simulink model "TEST_TCP"  (R2022b)
settings: Solver=FixedStepAuto  StartTime=0.0  StopTime=inf  FixedStep=1e-3  RelTol=1e-3  EnableMultiTasking=on
undefined symbols (not defined in the file or in its folder): angular, CIRCUIT, CLTF_DAMP, CLTF_FREQ, CLTF_GAIN, CONTROL, CONTROL_INI, DiscIntNeverNeededParam, INPUT, linear, MCP3201, MD25, MODEL, MODEL_INI, mpcstate, MPU60X0, MPU9250, MSG, NAV_MPC_CONTROL, OUTPUT, RCRX, SAMPLING_TIME, SYSID_INPUT, VL6180X
libraries: raspberrypiCommlib x156, simulink x86, dspsigattribs x14, raspberrypiNetworklib x13, embedlinuxBasiclib x9, ctrlSharedLib x2, ros2lib x2, mpclib x1, vrlib x1, sldrtlib x1
(part 5 of 17)

== system TEST_TCP/HARDWARE/SENSORS/IMU MPU60X0_SPI/READ FIFO ==
  Enable : EnablePort
  Constant2 : Constant  Commented=on  Value=bin2dec('01000100');  OutDataTypeStr=uint8  SampleTime=SAMPLING_TIME
  Constant3 : Constant  Value=MPU60X0.ACCEL_SSF  SampleTime=SAMPLING_TIME
  Constant4 : Constant  Value=MPU60X0.GYRO_SSF  SampleTime=SAMPLING_TIME
  Constant7 : Constant  Value=MPU60X0.FIFO_LENGTH  OutDataTypeStr=uint8  SampleTime=SAMPLING_TIME
  Data Store Read : DataStoreRead  DataStoreName=CONTROL  DataStoreElements=CONTROL_BUS.INPUT.IMU.ACCEL_MEAN(:,:)#CONTROL_BUS.INPUT.IMU.GYRO_MEAN(:,:)  IndexOptions=Index vector (dialog)  Indices=1  OutputSizes=1
  Data Store Read2 : DataStoreRead  DataStoreName=CONTROL  SampleTime=SAMPLING_TIME  IndexOptions=Index vector (dialog)  Indices=1  OutputSizes=1
  Data Store Write : DataStoreWrite  DataStoreName=CONTROL  IndexOptions=Index vector (dialog)  Indices=1  OutputSizes=1
  Data Store Write1 : DataStoreWrite  DataStoreName=MPU60X0_RAW_GYRO_MEAN  IndexOptions=Index vector (dialog)  Indices=1  OutputSizes=1
  Data Store Write2 : DataStoreWrite  DataStoreName=MPU60X0_RAW_ACCEL_MEAN  IndexOptions=Index vector (dialog)  Indices=1  OutputSizes=1
  Data Type Conversion : DataTypeConversion  OutDataTypeStr=double  SaturateOnIntegerOverflow=off  RndMeth=Floor
  Data Type Conversion4 : DataTypeConversion  OutDataTypeStr=int16  SaturateOnIntegerOverflow=off  RndMeth=Floor
  EVEN POSITIONS : Selector  InputPortWidth=uint8(12*MPU9250.FIFO_LENGTH)  IndexOptions=Index vector (dialog)  Indices=2:2:uint8(12*MPU9250.FIFO_LENGTH)  OutputSizes=1
  FIFO READ : Subsystem  mask{Register=MPU60X0.FIFO_R_W, n=12*MPU60X0.FIFO_LENGTH}
      mask prompts: Register "MPU9250 Register"; n "Data size (bytes)"
      mask DialogControl Control2 Prompt: (Add text here)
  FIFO RESET : raspberrypiCommlib/SPI Register Write  Priority=20  Commented=on  BoardProperty=Pi 3 Model B+  SSPin=SPI0_CE1  SPIModule=uint32(0)  Mode=Master  BusSpeed=1000000  Pin=SPI0_CE0  FirstBitToTransfer=Most significant bit (MSB)  ClockMode=3  BlockFunction=Write  RegisterAddress=MPU60X0.USER_CTRL  OutputDataType=int8  OutputDataLength=1
  FIFO_PROCESSING : MATLAB Function  Priority=30  TreatAsAtomicUnit=on
  Gain61 : Gain  Gain=2^8
  Mux : Mux
  ODD POSITIONS : Selector  InputPortWidth=uint8(12*MPU9250.FIFO_LENGTH)  IndexOptions=Index vector (dialog)  Indices=1:2:uint8(12*MPU9250.FIFO_LENGTH)  OutputSizes=1
  Sum61 : Sum  Inputs=|++
  To File : ToFile  Filename=BLACK_BOX_FIFO.mat  MatrixName=FIFO_LOG
  wires:
  Data Store Read/2 -> Mux/4
  Data Store Read/1 -> Mux/3
  FIFO_PROCESSING/5(GYRO_FIFO) -> Mux/2
  FIFO_PROCESSING/4(ACCEL_FIFO) -> Mux/1
  Constant4/1 -> FIFO_PROCESSING/5(GYRO_SSF)
  Constant3/1 -> FIFO_PROCESSING/4(ACCEL_SSF)
  Mux/1 -> Data Type Conversion/1
  Data Type Conversion/1 -> To File/1
  Data Type Conversion4/1 -> FIFO_PROCESSING/2(FIFO_DATA)
  FIFO READ/1(Out1) -> ODD POSITIONS/1, EVEN POSITIONS/1
  FIFO_PROCESSING/3(RAW_ACCEL_MEAN_OUT) -> Data Store Write2/1
  FIFO_PROCESSING/2(RAW_GYRO_MEAN_OUT) -> Data Store Write1/1
  Constant2/1 -> FIFO RESET/1
  Data Store Read2/1 -> FIFO_PROCESSING/1(CONTROL_IN)
  Sum61/1 -> Data Type Conversion4/1
  FIFO_PROCESSING/1(CONTROL_OUT) -> Data Store Write/1
  Constant7/1 -> FIFO_PROCESSING/3(FIFO_LENGTH)
  EVEN POSITIONS/1 -> Sum61/2
  Gain61/1 -> Sum61/1
  ODD POSITIONS/1 -> Gain61/1

== system TEST_TCP/HARDWARE/SENSORS/IMU MPU60X0_SPI/READ IMU ==
  Enable : EnablePort
  " LPF 3" : Subsystem
  " LPF 4" : Subsystem
  ACCELEROMETER : Subsystem  mask{REGISTER_ADDRESS=MPU60X0.ACCEL_XOUT_H, READ_FLAG=MPU60X0.READ_FLAG, N=6, Ts=MPU60X0.SAMPLING_TIME}
      mask prompts: REGISTER_ADDRESS "REGISTER ADDRESS"; READ_FLAG "READ FLAG"; N "DATA SIZE (BYTES)"; Ts "SAMPLING TIME (s)"
  Constant2 : Constant  Value=MPU60X0.ACCEL_CALIB  SampleTime=MPU60X0.SAMPLING_TIME
  Constant3 : Constant  Value=CONTROL_INI.PARAM.GRAVITY  SampleTime=MPU60X0.SAMPLING_TIME
  Constant4 : Constant  Value=MPU60X0.ALFA_CALIB  SampleTime=MPU60X0.SAMPLING_TIME
  Data Store Memory1 : DataStoreMemory  Priority=10  DataStoreName=MPU60X0_PITCH_OFFS  ReadBeforeWriteMsg=warning  WriteAfterWriteMsg=warning  WriteAfterReadMsg=warning  ShowAdditionalParam=off  OutDataTypeStr=double
  Data Store Memory5 : DataStoreMemory  Priority=10  DataStoreName=MPU60X0_ACCEL_OFFS  ReadBeforeWriteMsg=warning  WriteAfterWriteMsg=warning  WriteAfterReadMsg=warning  InitialValue=zeros(3,1)  ShowAdditionalParam=off  OutDataTypeStr=double
  Data Store Memory6 : DataStoreMemory  Priority=10  DataStoreName=MPU60X0_GYRO_OFFS  ReadBeforeWriteMsg=warning  WriteAfterWriteMsg=warning  WriteAfterReadMsg=warning  InitialValue=zeros(3,1)  ShowAdditionalParam=off  OutDataTypeStr=double
  Data Store Read : DataStoreRead  DataStoreName=CONTROL  SampleTime=MPU60X0.SAMPLING_TIME  DataStoreElements=CONTROL.STATE.VEHICLE_MODE  IndexOptions=Index vector (dialog)  Indices=1  OutputSizes=1
  Data Store Read1 : DataStoreRead  DataStoreName=MPU60X0_PITCH_OFFS  SampleTime=MPU60X0.SAMPLING_TIME  IndexOptions=Index vector (dialog)  Indices=1  OutputSizes=1
  Data Store Read6 : DataStoreRead  DataStoreName=MPU60X0_ACCEL_OFFS  SampleTime=MPU60X0.SAMPLING_TIME  IndexOptions=Index vector (dialog)  Indices=1  OutputSizes=1
  Data Store Read8 : DataStoreRead  DataStoreName=MPU60X0_GYRO_OFFS  SampleTime=MPU60X0.SAMPLING_TIME  IndexOptions=Index vector (dialog)  Indices=1  OutputSizes=1
  Data Store Read9 : DataStoreRead  DataStoreName=CONTROL  SampleTime=MPU60X0.SAMPLING_TIME  IndexOptions=Index vector (dialog)  Indices=1  OutputSizes=1
  Data Store Write3 : DataStoreWrite  DataStoreName=MPU60X0_ACCEL_OFFS  IndexOptions=Index vector (dialog)  Indices=1  OutputSizes=1
  Data Store Write4 : DataStoreWrite  DataStoreName=MPU60X0_GYRO_OFFS  IndexOptions=Index vector (dialog)  Indices=1  OutputSizes=1
  Data Store Write5 : DataStoreWrite  DataStoreName=CONTROL  IndexOptions=Index vector (dialog)  Indices=1  OutputSizes=1
  Data Type Conversion1 : DataTypeConversion  OutDataTypeStr=int16  SaturateOnIntegerOverflow=off  RndMeth=Floor
  Data Type Conversion2 : DataTypeConversion  OutDataTypeStr=double  SaturateOnIntegerOverflow=off  RndMeth=Floor
  Data Type Conversion3 : DataTypeConversion  OutDataTypeStr=double  SaturateOnIntegerOverflow=off  RndMeth=Floor
  Data Type Conversion4 : DataTypeConversion  OutDataTypeStr=int16  SaturateOnIntegerOverflow=off  RndMeth=Floor
  EVEN POSITIONS : Selector  InputPortWidth=uint8(6)  IndexOptions=Index vector (dialog)  Indices=2:2:uint8(6)  OutputSizes=1
  "EVEN POSITIONS  " : Selector  InputPortWidth=uint8(6)  IndexOptions=Index vector (dialog)  Indices=2:2:uint8(6)  OutputSizes=1
  FILTER POLE : Subsystem
  GRAVITY ROTATION : MATLAB Function  TreatAsAtomicUnit=on
  GYROSCOPE : Subsystem  mask{REGISTER_ADDRESS=MPU60X0.GYRO_XOUT_H, READ_FLAG=MPU60X0.READ_FLAG, N=6, Ts=MPU60X0.SAMPLING_TIME}
      mask prompts: REGISTER_ADDRESS "REGISTER ADDRESS"; READ_FLAG "READ FLAG"; N "DATA SIZE (BYTES)"; Ts "SAMPLING TIME (s)"
  Gain : Gain  Gain=CONTROL_INI.PARAM.GRAVITY/MPU60X0.ACCEL_SSF
  Gain1 : Gain  Gain=pi/MPU60X0.GYRO_SSF/180
  Gain4 : Gain  Gain=2^8
  Gain61 : Gain  Gain=2^8
  IMU CALIBRATION : MATLAB Function  Priority=30  TreatAsAtomicUnit=on
  LPF 1 : Subsystem
  "LPF 2 " : Subsystem
  MEAN FILTER : DiscreteFilter  Numerator=1/floor(SAMPLING_TIME*1000)*ones(1,floor(SAMPLING_TIME*1000))  Denominator=[1 zeros(1,floor(SAMPLING_TIME*1000)-1)]
  "MEAN FILTER " : DiscreteFilter  Numerator=1/floor(SAMPLING_TIME*1000)*ones(1,floor(SAMPLING_TIME*1000))  Denominator=[1 zeros(1,floor(SAMPLING_TIME*1000)-1)]
  ODD POSITIONS : Selector  InputPortWidth=uint8(6)  IndexOptions=Index vector (dialog)  Indices=1:2:uint8(6)  OutputSizes=1
  "ODD POSITIONS  " : Selector  InputPortWidth=uint8(6)  IndexOptions=Index vector (dialog)  Indices=1:2:uint8(6)  OutputSizes=1
  Sum4 : Sum  Inputs=|++
  Sum61 : Sum  Inputs=|++
  wires:
  ODD POSITIONS/1 -> Gain61/1
  EVEN POSITIONS/1 -> Sum61/2
  ACCELEROMETER/1(DATA_OUT) -> EVEN POSITIONS/1, ODD POSITIONS/1
  Sum61/1 -> Data Type Conversion4/1
  Gain61/1 -> Sum61/1
  Sum4/1 -> Data Type Conversion1/1
  Gain4/1 -> Sum4/1
  GYROSCOPE/1(DATA_OUT) -> "EVEN POSITIONS  "/1, "ODD POSITIONS  "/1
  "EVEN POSITIONS  "/1 -> Sum4/2
  "ODD POSITIONS  "/1 -> Gain4/1
  Data Type Conversion4/1 -> Data Type Conversion2/1
  Data Type Conversion1/1 -> Data Type Conversion3/1
  Data Type Conversion2/1 -> Gain/1
  Data Type Conversion3/1 -> Gain1/1
  Constant4/1 -> IMU CALIBRATION/11(ALFA_CALIB)
  Constant2/1 -> IMU CALIBRATION/10(ACCEL_CALIB)
  FILTER POLE/1(ALFA) -> " LPF 4"/2(ALFA), " LPF 3"/2(ALFA), LPF 1/2(ALFA), "LPF 2 "/2(ALFA)
  Gain1/1 -> "MEAN FILTER "/1, IMU CALIBRATION/6(GYRO), " LPF 3"/1(IN)
  LPF 1/1(OUT) -> IMU CALIBRATION/3(ACCEL_FILT)
  " LPF 3"/1(OUT) -> IMU CALIBRATION/7(GYRO_FILT)
  " LPF 4"/1(OUT) -> IMU CALIBRATION/9(GYRO_MEAN_FILT)
  Data Store Read9/1 -> IMU CALIBRATION/1(CONTROL_IN)
  "LPF 2 "/1(OUT) -> IMU CALIBRATION/5(ACCEL_MEAN_FILT)
  IMU CALIBRATION/3(GYRO_OFFS_OUT) -> Data Store Write4/1
  Data Store Read6/1 -> IMU CALIBRATION/12(ACCEL_OFFS_IN)
  IMU CALIBRATION/1(CONTROL) -> Data Store Write5/1
  MEAN FILTER/1 -> "LPF 2 "/1(IN), IMU CALIBRATION/4(ACCEL_MEAN)
  Data Store Read8/1 -> IMU CALIBRATION/13(GYRO_OFFS_IN)
  IMU CALIBRATION/2(ACCEL_OFFS_OUT) -> Data Store Write3/1
  "MEAN FILTER "/1 -> IMU CALIBRATION/8(GYRO_MEAN), " LPF 4"/1(IN)
  Gain/1 -> MEAN FILTER/1, IMU CALIBRATION/2(ACCEL), LPF 1/1(IN)
  Constant3/1 -> GRAVITY ROTATION/2(GRAVITY)
  Data Store Read1/1 -> GRAVITY ROTATION/1(PITCH_OFFSET)
  GRAVITY ROTATION/1(GRAVITY_VECTOR) -> IMU CALIBRATION/14(GRAVITY_VECTOR)
  Data Store Read/1 -> GRAVITY ROTATION/3(VEHICLE_MODE)

== system TEST_TCP/HARDWARE/SENSORS/IMU MPU60X0_SPI/READ TEMP ==
  Enable : EnablePort
  Bus Assignment : BusAssignment  AssignedSignals=INPUT.IMU.TEMP
  Constant1 : Constant  Value=MPU60X0.TEMP_SSF  SampleTime=MPU60X0.SAMPLING_TIME
  Constant2 : Constant  Value=MPU60X0.TEMP_OFFS  SampleTime=MPU60X0.SAMPLING_TIME
  Data Store Read1 : DataStoreRead  DataStoreName=CONTROL  SampleTime=MPU60X0.SAMPLING_TIME  IndexOptions=Index vector (dialog)  Indices=1  OutputSizes=1
  Data Store Read2 : DataStoreRead  DataStoreName=CONTROL  SampleTime=MPU60X0.SAMPLING_TIME  IndexOptions=Index vector (dialog)  Indices=1  OutputSizes=1
  Data Store Write : DataStoreWrite  DataStoreName=CONTROL  IndexOptions=Index vector (dialog)  Indices=1  OutputSizes=1
  Data Store Write1 : DataStoreWrite  DataStoreName=CONTROL  IndexOptions=Index vector (dialog)  Indices=1  OutputSizes=1
  Data Type Conversion3 : DataTypeConversion  OutDataTypeStr=int16  SaturateOnIntegerOverflow=off  RndMeth=Floor
  Demux : Demux  Outputs=2
  Gain61 : Gain  Gain=2^8
  IMU SCALING : MATLAB Function  Priority=40  TreatAsAtomicUnit=on
  Sum61 : Sum  Inputs=|++
  TEMP_READ : Subsystem  mask{REGISTER_ADDRESS=MPU60X0.TEMP_OUT_H, READ_FLAG=MPU60X0.READ_FLAG, N=2, Ts=MPU60X0.SAMPLING_TIME}
      mask prompts: REGISTER_ADDRESS "REGISTER ADDRESS"; READ_FLAG "READ FLAG"; N "DATA SIZE (BYTES)"; Ts "SAMPLING TIME (s)"
  wires:
  IMU SCALING/1(CONTROL_OUT) -> Data Store Write/1
  Demux/2 -> Sum61/2
  Sum61/1 -> Data Type Conversion3/1
  Bus Assignment/1 -> Data Store Write1/1
  Data Store Read1/1 -> Bus Assignment/1
  Gain61/1 -> Sum61/1
  Demux/1 -> Gain61/1
  Constant2/1 -> IMU SCALING/3(TEMP_OFFS)
  Data Type Conversion3/1 -> Bus Assignment/2
  Data Store Read2/1 -> IMU SCALING/1(CONTROL_IN)
  Constant1/1 -> IMU SCALING/2(TEMP_SSF)
  TEMP_READ/1(DATA_OUT) -> Demux/1

== system TEST_TCP/HARDWARE/SENSORS/IMU MPU60X0_SPI/WHO_AM_I ==
  Enable : EnablePort
  Display : Display
  MPU60X0_WHO_AM_I : Subsystem  Priority=10  mask{REGISTER_ADDRESS=MPU60X0.WHO_AM_I, READ_FLAG=MPU60X0.READ_FLAG, N=1, Ts=MPU60X0.SAMPLING_TIME}
      mask prompts: REGISTER_ADDRESS "REGISTER ADDRESS"; READ_FLAG "READ FLAG"; N "DATA SIZE (BYTES)"; Ts "SAMPLING TIME (s)"
  wires:
  MPU60X0_WHO_AM_I/1(DATA_OUT) -> Display/1

== system TEST_TCP/HARDWARE/SENSORS/WALL RANGE SENSOR/ANGLE AND DISTANCE COMPUTATION ==
  Data Store Read : DataStoreRead  DataStoreName=FRONT_DISTANCE  SampleTime=SAMPLING_TIME  IndexOptions=Index vector (dialog)  Indices=1  OutputSizes=1
  Data Store Read1 : DataStoreRead  DataStoreName=REAR_DISTANCE  IndexOptions=Index vector (dialog)  Indices=1  OutputSizes=1
  Data Store Read2 : DataStoreRead  DataStoreName=CONTROL  SampleTime=SAMPLING_TIME  IndexOptions=Index vector (dialog)  Indices=1  OutputSizes=1
  Data Store Write1 : DataStoreWrite  DataStoreName=CONTROL  IndexOptions=Index vector (dialog)  Indices=1  OutputSizes=1
  YAW_ANGLE_DISTANCE_COMPUTATION : MATLAB Function  TreatAsAtomicUnit=on
  wires:
  Data Store Read/1 -> YAW_ANGLE_DISTANCE_COMPUTATION/1(FRONT_DISTANCE)
  Data Store Read1/1 -> YAW_ANGLE_DISTANCE_COMPUTATION/2(REAR_DISTANCE)
  Data Store Read2/1 -> YAW_ANGLE_DISTANCE_COMPUTATION/3(CONTROL_IN)
  YAW_ANGLE_DISTANCE_COMPUTATION/1(CONTROL) -> Data Store Write1/1

== system TEST_TCP/HARDWARE/SENSORS/WALL RANGE SENSOR/VL6180X_I2C_FRONT ==
  Constant2 : Constant  Value=hex2dec('02')  OutDataTypeStr=uint8  SampleTime=SAMPLING_TIME
  Data Store Memory1 : DataStoreMemory  Priority=10  DataStoreName=VL6180X_COUNTER  ReadBeforeWriteMsg=warning  WriteAfterWriteMsg=warning  WriteAfterReadMsg=warning  ShowAdditionalParam=off  OutDataTypeStr=uint8
  Data Store Memory2 : DataStoreMemory  Priority=10  DataStoreName=VL6180X_RANGE_VAL  ReadBeforeWriteMsg=warning  WriteAfterWriteMsg=warning  WriteAfterReadMsg=warning  ShowAdditionalParam=off  OutDataTypeStr=uint8
  Data Store Memory3 : DataStoreMemory  Priority=10  DataStoreName=VL6180X_STATUS  ReadBeforeWriteMsg=warning  WriteAfterWriteMsg=warning  WriteAfterReadMsg=warning  ShowAdditionalParam=off  OutDataTypeStr=uint8
  Data Store Read : DataStoreRead  Priority=30  DataStoreName=VL6180X_RANGE_VAL  SampleTime=SAMPLING_TIME  IndexOptions=Index vector (dialog)  Indices=1  OutputSizes=1
  Data Store Read2 : DataStoreRead  DataStoreName=VL6180X_STATUS  SampleTime=SAMPLING_TIME  IndexOptions=Index vector (dialog)  Indices=1  OutputSizes=1
  Data Store Write : DataStoreWrite  DataStoreName=FRONT_DISTANCE  IndexOptions=Index vector (dialog)  Indices=1  OutputSizes=1
  Data Type Conversion : DataTypeConversion  OutDataTypeStr=double  SaturateOnIntegerOverflow=off  RndMeth=Floor
  I2C MULTIPLEXER WRITE : raspberrypiCommlib/I2C Master Write  Priority=5  BoardProperty=Pi 3 Model B+  Mode=Master  SlaveAddress=hex2dec('70')  SlaveByteOrder=BigEndian  Direction=Transmitter  RegisterAddressMode=off  RegisterAddress=hex2dec('207')  SlaveDataType=uint8  DataLength=1  NoAck=off  RepeatedStart=off  OutputStatus=off
  INITIALIZATION : simulink/Logic and Bit Operations/Compare To Constant  relop===  const=0  OutDataTypeStr=boolean
  MEASUREMENT : simulink/Logic and Bit Operations/Compare To Constant  relop===  const=1  OutDataTypeStr=boolean
  READ RANGE : Subsystem  Priority=20
  VL6180X INITIALIZATION : Subsystem  Priority=10
      settings: RTWSystemCode=Nonreusable function
  wires:
  INITIALIZATION/1 -> VL6180X INITIALIZATION/Enable
  Data Store Read2/1 -> MEASUREMENT/1, INITIALIZATION/1
  MEASUREMENT/1 -> READ RANGE/Enable
  Data Store Read/1 -> Data Type Conversion/1
  Constant2/1 -> I2C MULTIPLEXER WRITE/1
  Data Type Conversion/1 -> Data Store Write/1

== system TEST_TCP/HARDWARE/SENSORS/WALL RANGE SENSOR/VL6180X_I2C_REAR ==
  Constant2 : Constant  Value=hex2dec('01')  OutDataTypeStr=uint8  SampleTime=SAMPLING_TIME
  Data Store Memory1 : DataStoreMemory  Priority=10  DataStoreName=VL6180X_COUNTER  ReadBeforeWriteMsg=warning  WriteAfterWriteMsg=warning  WriteAfterReadMsg=warning  ShowAdditionalParam=off  OutDataTypeStr=uint8
  Data Store Memory2 : DataStoreMemory  Priority=10  DataStoreName=VL6180X_RANGE_VAL  ReadBeforeWriteMsg=warning  WriteAfterWriteMsg=warning  WriteAfterReadMsg=warning  ShowAdditionalParam=off  OutDataTypeStr=uint8
  Data Store Memory3 : DataStoreMemory  Priority=10  DataStoreName=VL6180X_STATUS  ReadBeforeWriteMsg=warning  WriteAfterWriteMsg=warning  WriteAfterReadMsg=warning  ShowAdditionalParam=off  OutDataTypeStr=uint8
  Data Store Read : DataStoreRead  Priority=30  DataStoreName=VL6180X_RANGE_VAL  SampleTime=SAMPLING_TIME  IndexOptions=Index vector (dialog)  Indices=1  OutputSizes=1
  Data Store Read2 : DataStoreRead  DataStoreName=VL6180X_STATUS  SampleTime=SAMPLING_TIME  IndexOptions=Index vector (dialog)  Indices=1  OutputSizes=1
  Data Store Write : DataStoreWrite  DataStoreName=REAR_DISTANCE  IndexOptions=Index vector (dialog)  Indices=1  OutputSizes=1
  Data Type Conversion : DataTypeConversion  OutDataTypeStr=double  SaturateOnIntegerOverflow=off  RndMeth=Floor
  I2C MULTIPLEXER WRITE : raspberrypiCommlib/I2C Master Write  Priority=5  BoardProperty=Pi 3 Model B+  Mode=Master  SlaveAddress=hex2dec('70')  SlaveByteOrder=BigEndian  Direction=Transmitter  RegisterAddressMode=off  RegisterAddress=hex2dec('207')  SlaveDataType=uint8  DataLength=1  NoAck=off  RepeatedStart=off  OutputStatus=off
  INITIALIZATION : simulink/Logic and Bit Operations/Compare To Constant  relop===  const=0  OutDataTypeStr=boolean
  MEASUREMENT : simulink/Logic and Bit Operations/Compare To Constant  relop===  const=1  OutDataTypeStr=boolean
  READ RANGE : Subsystem  Priority=20
  VL6180X INITIALIZATION : Subsystem  Priority=10
      settings: RTWSystemCode=Nonreusable function
  wires:
  Constant2/1 -> I2C MULTIPLEXER WRITE/1
  Data Store Read/1 -> Data Type Conversion/1
  MEASUREMENT/1 -> READ RANGE/Enable
  Data Store Read2/1 -> INITIALIZATION/1, MEASUREMENT/1
  INITIALIZATION/1 -> VL6180X INITIALIZATION/Enable
  Data Type Conversion/1 -> Data Store Write/1

== system TEST_TCP/HARDWARE/SENSORS/IMU MPU60X0_SPI/INITIALIZATION/Subsystem ==
  Constant3 : Constant  Value=Register  OutDataTypeStr=uint8  SampleTime=-1
  Constant4 : Constant  Value=MPU60X0.READ_FLAG  OutDataTypeStr=uint8  SampleTime=-1
  Constant5 : Constant  Value=zeros(n,1)  OutDataTypeStr=uint8  SampleTime=-1
  Demux : Demux  Outputs=[1 -1]
  Mux : Mux  Inputs=2
  SPI Master Transfer : raspberrypiCommlib/SPI Master Transfer  BoardProperty=Pi 3 Model B+  SSPin=SPI0_CE1  SPIModule=uint32(0)  Mode=Master  BusSpeed=1000000  Pin=SPI0_CE0  FirstBitToTransfer=Most significant bit (MSB)  ClockMode=3  BlockFunction=Transfer  RegisterAddress=0  OutputDataType=int8  OutputDataLength=1
  Sum : Sum  Inputs=|++
  Terminator : Terminator
  Out1 : Outport  VectorParamsAs1DForOutWhenUnconnected=off
  wires:
  Constant5/1 -> Mux/2
  Constant4/1 -> Sum/2
  Mux/1 -> SPI Master Transfer/1
  Demux/2 -> Out1/1
  Sum/1 -> Mux/1
  SPI Master Transfer/1 -> Demux/1
  Demux/1 -> Terminator/1
  Constant3/1 -> Sum/1

== system TEST_TCP/HARDWARE/SENSORS/IMU MPU60X0_SPI/READ FIFO/FIFO READ ==
  Constant3 : Constant  Value=Register  OutDataTypeStr=uint8  SampleTime=SAMPLING_TIME
  Constant4 : Constant  Value=MPU9250.READ_FLAG  OutDataTypeStr=uint8  SampleTime=-1
  Constant5 : Constant  Value=zeros(n,1)  OutDataTypeStr=uint8  SampleTime=-1
  Demux : Demux  Outputs=[1 -1]
  Mux : Mux  Inputs=2
  SPI Master Transfer : raspberrypiCommlib/SPI Master Transfer  BoardProperty=Pi 3 Model B+  SSPin=SPI0_CE1  SPIModule=uint32(0)  Mode=Master  BusSpeed=1000000  Pin=SPI0_CE1  FirstBitToTransfer=Most significant bit (MSB)  ClockMode=3  BlockFunction=Transfer  RegisterAddress=0  OutputDataType=int8  OutputDataLength=1
  Sum : Sum  Inputs=|++
  Terminator : Terminator
  Out1 : Outport  VectorParamsAs1DForOutWhenUnconnected=off
  wires:
  Constant5/1 -> Mux/2
  Constant4/1 -> Sum/2
  Mux/1 -> SPI Master Transfer/1
  Demux/2 -> Out1/1
  Sum/1 -> Mux/1
  SPI Master Transfer/1 -> Demux/1
  Demux/1 -> Terminator/1
  Constant3/1 -> Sum/1

== system TEST_TCP/HARDWARE/SENSORS/IMU MPU60X0_SPI/READ IMU/ LPF 3 ==
  IN : Inport
  ALFA : Inport  Port=2  SampleTime=MPU60X0.SAMPLING_TIME
  Bias : Bias  Bias=1  SaturateOnIntegerOverflow=off
  Gain : Gain  Gain=-1
  Product : Product
  Product2 : Product
  Sum : Sum  Inputs=|++
  Unit Delay : UnitDelay  SampleTime=-1  HasFrameUpgradeWarning=on
  OUT : Outport  VectorParamsAs1DForOutWhenUnconnected=off
  wires:
  IN/1 -> Product2/1
  Bias/1 -> Product2/2
  Product2/1 -> Sum/1
  Gain/1 -> Bias/1
  ALFA/1 -> Product/2, Gain/1
  Sum/1 -> OUT/1, Unit Delay/1
  Product/1 -> Sum/2
  Unit Delay/1 -> Product/1

== system TEST_TCP/HARDWARE/SENSORS/IMU MPU60X0_SPI/READ IMU/ LPF 4 ==
  IN : Inport
  ALFA : Inport  Port=2  SampleTime=MPU60X0.SAMPLING_TIME
  Bias : Bias  Bias=1  SaturateOnIntegerOverflow=off
  Gain : Gain  Gain=-1
  Product : Product
  Product2 : Product
  Sum : Sum  Inputs=|++
  Unit Delay : UnitDelay  SampleTime=-1  HasFrameUpgradeWarning=on
  OUT : Outport  VectorParamsAs1DForOutWhenUnconnected=off
  wires:
  IN/1 -> Product2/1
  Bias/1 -> Product2/2
  Product2/1 -> Sum/1
  Gain/1 -> Bias/1
  ALFA/1 -> Product/2, Gain/1
  Sum/1 -> OUT/1, Unit Delay/1
  Product/1 -> Sum/2
  Unit Delay/1 -> Product/1

== system TEST_TCP/HARDWARE/SENSORS/IMU MPU60X0_SPI/READ IMU/ACCELEROMETER ==
  Constant3 : Constant  Value=REGISTER_ADDRESS  OutDataTypeStr=uint8  SampleTime=Ts
  Constant4 : Constant  Value=READ_FLAG  OutDataTypeStr=uint8  SampleTime=Ts
  Constant5 : Constant  Value=zeros(N,1)  OutDataTypeStr=uint8  SampleTime=Ts
  Demux : Demux  Outputs=[1 -1]
  Mux : Mux  Inputs=2
  SPI Master Transfer : raspberrypiCommlib/SPI Master Transfer  BoardProperty=Pi 3 Model B+  SSPin=SPI0_CE1  SPIModule=uint32(0)  Mode=Master  BusSpeed=1000000  Pin=SPI0_CE0  FirstBitToTransfer=Most significant bit (MSB)  ClockMode=3  BlockFunction=Transfer  RegisterAddress=0  OutputDataType=int8  OutputDataLength=1
  Sum : Sum  Inputs=|++
  Terminator : Terminator
  DATA_OUT : Outport  VectorParamsAs1DForOutWhenUnconnected=off
  wires:
  Constant3/1 -> Sum/1
  Demux/1 -> Terminator/1
  SPI Master Transfer/1 -> Demux/1
  Sum/1 -> Mux/1
  Demux/2 -> DATA_OUT/1
  Mux/1 -> SPI Master Transfer/1
  Constant4/1 -> Sum/2
  Constant5/1 -> Mux/2

== system TEST_TCP/HARDWARE/SENSORS/IMU MPU60X0_SPI/READ IMU/FILTER POLE ==
  Constant : Constant  Value=MPU60X0.SAMPLING_TIME  OutDataTypeStr=single  SampleTime=MPU60X0.SAMPLING_TIME
  Data Store Read4 : DataStoreRead  DataStoreName=CONTROL  SampleTime=MPU60X0.SAMPLING_TIME  DataStoreElements=CONTROL.PARAM.IMU_FILT_FREQ  IndexOptions=Index vector (dialog)  Indices=1  OutputSizes=1
  Gain : Gain  Gain=-2*pi
  Math Function : Math  SignedPower=on
  Product1 : Product
  ALFA : Outport  VectorParamsAs1DForOutWhenUnconnected=off
  wires:
  Data Store Read4/1 -> Gain/1
  Product1/1 -> Math Function/1
  Constant/1 -> Product1/1
  Math Function/1 -> ALFA/1
  Gain/1 -> Product1/2

== system TEST_TCP/HARDWARE/SENSORS/IMU MPU60X0_SPI/READ IMU/GYROSCOPE ==
  Constant3 : Constant  Value=REGISTER_ADDRESS  OutDataTypeStr=uint8  SampleTime=Ts
  Constant4 : Constant  Value=READ_FLAG  OutDataTypeStr=uint8  SampleTime=Ts
  Constant5 : Constant  Value=zeros(N,1)  OutDataTypeStr=uint8  SampleTime=Ts
  Demux : Demux  Outputs=[1 -1]
  Mux : Mux  Inputs=2
  SPI Master Transfer : raspberrypiCommlib/SPI Master Transfer  BoardProperty=Pi 3 Model B+  SSPin=SPI0_CE1  SPIModule=uint32(0)  Mode=Master  BusSpeed=1000000  Pin=SPI0_CE0  FirstBitToTransfer=Most significant bit (MSB)  ClockMode=3  BlockFunction=Transfer  RegisterAddress=0  OutputDataType=int8  OutputDataLength=1
  Sum : Sum  Inputs=|++
  Terminator : Terminator
  DATA_OUT : Outport  VectorParamsAs1DForOutWhenUnconnected=off
  wires:
  Constant5/1 -> Mux/2
  Constant4/1 -> Sum/2
  Mux/1 -> SPI Master Transfer/1
  Demux/2 -> DATA_OUT/1
  Sum/1 -> Mux/1
  SPI Master Transfer/1 -> Demux/1
  Demux/1 -> Terminator/1
  Constant3/1 -> Sum/1

== system TEST_TCP/HARDWARE/SENSORS/IMU MPU60X0_SPI/READ IMU/LPF 1 ==
  IN : Inport
  ALFA : Inport  Port=2  SampleTime=MPU60X0.SAMPLING_TIME
  Bias : Bias  Bias=1  SaturateOnIntegerOverflow=off
  Gain : Gain  Gain=-1
  Product : Product
  Product2 : Product
  Sum : Sum  Inputs=|++
  Unit Delay : UnitDelay  InitialCondition=[CONTROL_INI.PARAM.GRAVITY*CONTROL_INI.STATE.VEHICLE_MODE ; 0 ; -CONTROL_INI.PARAM.GRAVITY*(1-CONTROL_INI.STATE.VEHICLE_MODE)]  SampleTime=-1  HasFrameUpgradeWarning=on
  OUT : Outport  VectorParamsAs1DForOutWhenUnconnected=off
  wires:
  Unit Delay/1 -> Product/1
  Product/1 -> Sum/2
  Sum/1 -> Unit Delay/1, OUT/1
  ALFA/1 -> Gain/1, Product/2
  Gain/1 -> Bias/1
  Product2/1 -> Sum/1
  Bias/1 -> Product2/2
  IN/1 -> Product2/1

== system TEST_TCP/HARDWARE/SENSORS/IMU MPU60X0_SPI/READ IMU/LPF 2  ==
  IN : Inport
  ALFA : Inport  Port=2  SampleTime=MPU60X0.SAMPLING_TIME
  Bias : Bias  Bias=1  SaturateOnIntegerOverflow=off
  Gain : Gain  Gain=-1
  Product : Product
  Product2 : Product
  Sum : Sum  Inputs=|++
  Unit Delay : UnitDelay  InitialCondition=[CONTROL_INI.PARAM.GRAVITY*CONTROL_INI.STATE.VEHICLE_MODE ; 0 ; -CONTROL_INI.PARAM.GRAVITY*(1-CONTROL_INI.STATE.VEHICLE_MODE)]  SampleTime=-1  HasFrameUpgradeWarning=on
  OUT : Outport  VectorParamsAs1DForOutWhenUnconnected=off
  wires:
  Unit Delay/1 -> Product/1
  Product/1 -> Sum/2
  Sum/1 -> Unit Delay/1, OUT/1
  ALFA/1 -> Gain/1, Product/2
  Gain/1 -> Bias/1
  Product2/1 -> Sum/1
  Bias/1 -> Product2/2
  IN/1 -> Product2/1

== system TEST_TCP/HARDWARE/SENSORS/IMU MPU60X0_SPI/READ TEMP/TEMP_READ ==
  Constant3 : Constant  Value=REGISTER_ADDRESS  OutDataTypeStr=uint8  SampleTime=Ts
  Constant4 : Constant  Value=READ_FLAG  OutDataTypeStr=uint8  SampleTime=Ts
  Constant5 : Constant  Value=zeros(N,1)  OutDataTypeStr=uint8  SampleTime=Ts
  Demux : Demux  Outputs=[1 -1]
  Mux : Mux  Inputs=2
  SPI Master Transfer : raspberrypiCommlib/SPI Master Transfer  BoardProperty=Pi 3 Model B+  SSPin=SPI0_CE1  SPIModule=uint32(0)  Mode=Master  BusSpeed=1000000  Pin=SPI0_CE1  FirstBitToTransfer=Most significant bit (MSB)  ClockMode=3  BlockFunction=Transfer  RegisterAddress=0  OutputDataType=int8  OutputDataLength=1
  Sum : Sum  Inputs=|++
  Terminator : Terminator
  DATA_OUT : Outport  VectorParamsAs1DForOutWhenUnconnected=off
  wires:
  Constant5/1 -> Mux/2
  Constant4/1 -> Sum/2
  Mux/1 -> SPI Master Transfer/1
  Demux/2 -> DATA_OUT/1
  Sum/1 -> Mux/1
  SPI Master Transfer/1 -> Demux/1
  Demux/1 -> Terminator/1
  Constant3/1 -> Sum/1

== system TEST_TCP/HARDWARE/SENSORS/IMU MPU60X0_SPI/WHO_AM_I/MPU60X0_WHO_AM_I ==
  Constant3 : Constant  Value=REGISTER_ADDRESS  OutDataTypeStr=uint8  SampleTime=Ts
  Constant4 : Constant  Value=READ_FLAG  OutDataTypeStr=uint8  SampleTime=Ts
  Constant5 : Constant  Value=zeros(N,1)  OutDataTypeStr=uint8  SampleTime=Ts
  Demux : Demux  Outputs=[1 -1]
  Mux : Mux  Inputs=2
  SPI Master Transfer : raspberrypiCommlib/SPI Master Transfer  BoardProperty=Pi 3 Model B+  SSPin=SPI0_CE1  SPIModule=uint32(0)  Mode=Master  BusSpeed=1000000  Pin=SPI0_CE0  FirstBitToTransfer=Most significant bit (MSB)  ClockMode=3  BlockFunction=Transfer  RegisterAddress=0  OutputDataType=int8  OutputDataLength=1
  Sum : Sum  Inputs=|++
  Terminator : Terminator
  DATA_OUT : Outport  VectorParamsAs1DForOutWhenUnconnected=off
  wires:
  Constant3/1 -> Sum/1
  Demux/1 -> Terminator/1
  SPI Master Transfer/1 -> Demux/1
  Sum/1 -> Mux/1
  Demux/2 -> DATA_OUT/1
  Mux/1 -> SPI Master Transfer/1
  Constant4/1 -> Sum/2
  Constant5/1 -> Mux/2

== system TEST_TCP/HARDWARE/SENSORS/WALL RANGE SENSOR/VL6180X_I2C_FRONT/READ RANGE ==
  Enable : EnablePort
  Bitwise Operator : simulink/Logic and Bit Operations/Bitwise Operator  logicop=AND  UseBitMask=on  BitMask=hex2dec('04')  BitMaskRealWorld=Stored Integer
  CHECK READOUT : Subsystem  Priority=20
  Compare To Constant : simulink/Logic and Bit Operations/Compare To Constant  relop===  const=4  OutDataTypeStr=boolean
  I2C READ: RESULT_INTERRUPT_STATUS_GPIO : Subsystem  Priority=10  mask{SLAVE_ADDRESS=VL6180X.ADDRESS, REGISTER_ADDRESS=VL6180X.RESULT_INTERRUPT_STATUS_GPIO, N=1}
      mask prompts: SLAVE_ADDRESS "SLAVE ADDRESS"; REGISTER_ADDRESS "REGISTER ADDRESS"; N "NUMBER OF DATA (bytes)"
  Logical Operator : Logic  Operator=NOT  AllPortsSameDT=off  OutDataTypeStr=boolean
  READ RANGE VALUE : Subsystem  Priority=20
  READY1 : Constant  Value=VL6180X.RANGING_MODE  OutDataTypeStr=uint8  SampleTime=SAMPLING_TIME
  SINGLE_SHOT : simulink/Logic and Bit Operations/Compare To Constant  relop===  const=0  OutDataTypeStr=boolean
  START READ RANGE SINGLE : Subsystem  Priority=30  TreatAsAtomicUnit=on
      settings: RTWSystemCode=Nonreusable function
  wires:
  Bitwise Operator/1 -> Compare To Constant/1
  Compare To Constant/1 -> Logical Operator/1, READ RANGE VALUE/Enable
  I2C READ: RESULT_INTERRUPT_STATUS_GPIO/1(DATA) -> Bitwise Operator/1
  READY1/1 -> SINGLE_SHOT/1
  SINGLE_SHOT/1 -> START READ RANGE SINGLE/Enable
  Logical Operator/1 -> CHECK READOUT/Enable

== system TEST_TCP/HARDWARE/SENSORS/WALL RANGE SENSOR/VL6180X_I2C_FRONT/VL6180X INITIALIZATION ==
  note: Initialize sensor with settings from ST application note AN4545, section 9
  Enable : EnablePort
  CHECK INITIALIZATION : Subsystem  Priority=60
  Compare To Constant : simulink/Logic and Bit Operations/Compare To Constant  relop===  const=1  OutDataTypeStr=boolean
  Compare To Constant1 : simulink/Logic and Bit Operations/Compare To Constant  relop===  const=1  OutDataTypeStr=boolean
  I2C READ: SYSTEM_FRESH_OUT_OF_RESET : Subsystem  Priority=10  mask{SLAVE_ADDRESS=VL6180X.ADDRESS, REGISTER_ADDRESS=VL6180X.SYSTEM_FRESH_OUT_OF_RESET, N=1}
      mask prompts: SLAVE_ADDRESS "SLAVE ADDRESS"; REGISTER_ADDRESS "REGISTER ADDRESS"; N "NUMBER OF DATA (bytes)"
  LOAD PRIVATE REGISTERS (MANDATORY) : Subsystem  Priority=20
  LOAD PUBLIC REGISTERS (OPTIONAL) : Subsystem  Priority=40
      settings: RTWSystemCode=Nonreusable function
  LOAD PUBLIC REGISTERS (RECOMMENDED) : Subsystem  Priority=30
      settings: RTWSystemCode=Nonreusable function
  MEASUREMENT CONFIGURATION : Subsystem  Priority=70
      settings: RTWSystemCode=Nonreusable function
  OTHER SPECIFIC SETTINGS (OPTIONAL) : Subsystem  Priority=50
      settings: RTWSystemCode=Nonreusable function
  wires:
  Compare To Constant/1 -> OTHER SPECIFIC SETTINGS (OPTIONAL)/Enable, LOAD PUBLIC REGISTERS (OPTIONAL)/Enable, LOAD PUBLIC REGISTERS (RECOMMENDED)/Enable, LOAD PRIVATE REGISTERS (MANDATORY)/Enable
  I2C READ: SYSTEM_FRESH_OUT_OF_RESET/1(DATA) -> Compare To Constant/1
  CHECK INITIALIZATION/1(STATUS) -> Compare To Constant1/1
  Compare To Constant1/1 -> MEASUREMENT CONFIGURATION/Enable

== system TEST_TCP/HARDWARE/SENSORS/WALL RANGE SENSOR/VL6180X_I2C_REAR/READ RANGE ==
  Enable : EnablePort
  Bitwise Operator : simulink/Logic and Bit Operations/Bitwise Operator  logicop=AND  UseBitMask=on  BitMask=hex2dec('04')  BitMaskRealWorld=Stored Integer
  CHECK READOUT : Subsystem  Priority=20
  Compare To Constant : simulink/Logic and Bit Operations/Compare To Constant  relop===  const=4  OutDataTypeStr=boolean
  I2C READ: RESULT_INTERRUPT_STATUS_GPIO : Subsystem  Priority=10  mask{SLAVE_ADDRESS=VL6180X.ADDRESS, REGISTER_ADDRESS=VL6180X.RESULT_INTERRUPT_STATUS_GPIO, N=1}
      mask prompts: SLAVE_ADDRESS "SLAVE ADDRESS"; REGISTER_ADDRESS "REGISTER ADDRESS"; N "NUMBER OF DATA (bytes)"
  Logical Operator : Logic  Operator=NOT  AllPortsSameDT=off  OutDataTypeStr=boolean
  READ RANGE VALUE : Subsystem  Priority=20
  READY1 : Constant  Value=VL6180X.RANGING_MODE  OutDataTypeStr=uint8  SampleTime=SAMPLING_TIME
  SINGLE_SHOT : simulink/Logic and Bit Operations/Compare To Constant  relop===  const=0  OutDataTypeStr=boolean
  START READ RANGE SINGLE : Subsystem  Priority=30  TreatAsAtomicUnit=on
      settings: RTWSystemCode=Nonreusable function
  wires:
  Logical Operator/1 -> CHECK READOUT/Enable
  SINGLE_SHOT/1 -> START READ RANGE SINGLE/Enable
  READY1/1 -> SINGLE_SHOT/1
  I2C READ: RESULT_INTERRUPT_STATUS_GPIO/1(DATA) -> Bitwise Operator/1
  Compare To Constant/1 -> READ RANGE VALUE/Enable, Logical Operator/1
  Bitwise Operator/1 -> Compare To Constant/1

== system TEST_TCP/HARDWARE/SENSORS/WALL RANGE SENSOR/VL6180X_I2C_REAR/VL6180X INITIALIZATION ==
  note: Initialize sensor with settings from ST application note AN4545, section 9
  Enable : EnablePort
  CHECK INITIALIZATION : Subsystem  Priority=60
  Compare To Constant : simulink/Logic and Bit Operations/Compare To Constant  relop===  const=1  OutDataTypeStr=boolean
  Compare To Constant1 : simulink/Logic and Bit Operations/Compare To Constant  relop===  const=1  OutDataTypeStr=boolean
  I2C READ: SYSTEM_FRESH_OUT_OF_RESET : Subsystem  Priority=10  mask{SLAVE_ADDRESS=VL6180X.ADDRESS, REGISTER_ADDRESS=VL6180X.SYSTEM_FRESH_OUT_OF_RESET, N=1}
      mask prompts: SLAVE_ADDRESS "SLAVE ADDRESS"; REGISTER_ADDRESS "REGISTER ADDRESS"; N "NUMBER OF DATA (bytes)"
  LOAD PRIVATE REGISTERS (MANDATORY) : Subsystem  Priority=20
  LOAD PUBLIC REGISTERS (OPTIONAL) : Subsystem  Priority=40
      settings: RTWSystemCode=Nonreusable function
  LOAD PUBLIC REGISTERS (RECOMMENDED) : Subsystem  Priority=30
      settings: RTWSystemCode=Nonreusable function
  MEASUREMENT CONFIGURATION : Subsystem  Priority=70
      settings: RTWSystemCode=Nonreusable function
  OTHER SPECIFIC SETTINGS (OPTIONAL) : Subsystem  Priority=50
      settings: RTWSystemCode=Nonreusable function
  wires:
  Compare To Constant1/1 -> MEASUREMENT CONFIGURATION/Enable
  CHECK INITIALIZATION/1(STATUS) -> Compare To Constant1/1
  I2C READ: SYSTEM_FRESH_OUT_OF_RESET/1(DATA) -> Compare To Constant/1
  Compare To Constant/1 -> LOAD PRIVATE REGISTERS (MANDATORY)/Enable, LOAD PUBLIC REGISTERS (RECOMMENDED)/Enable, LOAD PUBLIC REGISTERS (OPTIONAL)/Enable, OTHER SPECIFIC SETTINGS (OPTIONAL)/Enable

== system TEST_TCP/HARDWARE/SENSORS/WALL RANGE SENSOR/VL6180X_I2C_FRONT/READ RANGE/CHECK READOUT ==
  Enable : EnablePort
  Bias : Bias  Bias=1  SaturateOnIntegerOverflow=off
  Compare To Constant : simulink/Logic and Bit Operations/Compare To Constant  relop=>=  const=20  OutDataTypeStr=boolean
  Data Store Read1 : DataStoreRead  DataStoreName=VL6180X_COUNTER  SampleTime=SAMPLING_TIME  IndexOptions=Index vector (dialog)  Indices=1  OutputSizes=1
  Data Store Write : DataStoreWrite  DataStoreName=VL6180X_COUNTER  IndexOptions=Index vector (dialog)  Indices=1  OutputSizes=1
  SENSOR INITIALIZATION : Subsystem
  wires:
  Data Store Read1/1 -> Bias/1
  Bias/1 -> Compare To Constant/1, Data Store Write/1
  Compare To Constant/1 -> SENSOR INITIALIZATION/Enable

== system TEST_TCP/HARDWARE/SENSORS/WALL RANGE SENSOR/VL6180X_I2C_FRONT/READ RANGE/I2C READ: RESULT_INTERRUPT_STATUS_GPIO ==
  Constant : Constant  Value=REGISTER_ADDRESS  OutDataTypeStr=uint16  SampleTime=SAMPLING_TIME
  DATA TO BE READ : raspberrypiCommlib/I2C Master Read  Priority=20  BoardProperty=Pi 3 Model B  Mode=Master  SlaveAddress=SLAVE_ADDRESS  SlaveByteOrder=BigEndian  Direction=Receiver  RegisterAddressMode=off  RegisterAddress=0  SlaveDataType=uint8  DataLength=uint8(N)  NoAck=off  RepeatedStart=off  OutputStatus=off  SampleTime=SAMPLING_TIME
  REGISTER ADDRESS : raspberrypiCommlib/I2C Master Write  Priority=10  BoardProperty=Pi 3 Model B  Mode=Master  SlaveAddress=SLAVE_ADDRESS  SlaveByteOrder=BigEndian  Direction=Transmitter  RegisterAddressMode=off  RegisterAddress=hex2dec('207')  SlaveDataType=uint8  DataLength=1  NoAck=off  RepeatedStart=off  OutputStatus=off
  DATA : Outport  VectorParamsAs1DForOutWhenUnconnected=off
  wires:
  DATA TO BE READ/1 -> DATA/1
  Constant/1 -> REGISTER ADDRESS/1

== system TEST_TCP/HARDWARE/SENSORS/WALL RANGE SENSOR/VL6180X_I2C_FRONT/READ RANGE/READ RANGE VALUE ==
  Enable : EnablePort
  Constant1 : Constant  Value=hex2dec('07')  OutDataTypeStr=uint8  SampleTime=SAMPLING_TIME
  Data Store Write : DataStoreWrite  DataStoreName=VL6180X_RANGE_VAL  IndexOptions=Index vector (dialog)  Indices=1  OutputSizes=1
  Data Store Write1 : DataStoreWrite  DataStoreName=VL6180X_COUNTER  IndexOptions=Index vector (dialog)  Indices=1  OutputSizes=1
  I2C READ: VL6180X.RESULT_RANGE_VAL : Subsystem  Priority=10  mask{SLAVE_ADDRESS=VL6180X.ADDRESS, REGISTER_ADDRESS=VL6180X.RESULT_RANGE_VAL, N=1}
      mask prompts: SLAVE_ADDRESS "SLAVE ADDRESS"; REGISTER_ADDRESS "REGISTER ADDRESS"; N "NUMBER OF DATA (bytes)"
  I2C WRITE: SYSTEM_INTERRUPT_CLEAR : Subsystem  Priority=20  mask{SLAVE_ADDRESS=VL6180X.ADDRESS, REGISTER_ADDRESS=VL6180X.SYSTEM_INTERRUPT_CLEAR}
      mask prompts: SLAVE_ADDRESS "SLAVE ADDRESS"; REGISTER_ADDRESS "REGISTER ADDRESS"
      mask init:
      | REGISTER_ADDRESS_MSB = uint8(floor(REGISTER_ADDRESS/(2^8)));
      | REGISTER_ADDRESS_LSB = uint8(rem(REGISTER_ADDRESS,2^8));
  READY1 : Constant  Value=0  OutDataTypeStr=uint8  SampleTime=SAMPLING_TIME
  wires:
  I2C READ: VL6180X.RESULT_RANGE_VAL/1(DATA) -> Data Store Write/1
  Constant1/1 -> I2C WRITE: SYSTEM_INTERRUPT_CLEAR/1(DATA)
  READY1/1 -> Data Store Write1/1

== system TEST_TCP/HARDWARE/SENSORS/WALL RANGE SENSOR/VL6180X_I2C_FRONT/READ RANGE/START READ RANGE SINGLE ==
  Enable : EnablePort
  Constant1 : Constant  Value=hex2dec('01')  OutDataTypeStr=uint8  SampleTime=SAMPLING_TIME
  I2C WRITE: SYSRANGE_START : Subsystem  mask{SLAVE_ADDRESS=VL6180X.ADDRESS, REGISTER_ADDRESS=VL6180X.SYSRANGE_START}
      mask prompts: SLAVE_ADDRESS "SLAVE ADDRESS"; REGISTER_ADDRESS "REGISTER ADDRESS"
      mask init:
      | REGISTER_ADDRESS_MSB = uint8(floor(REGISTER_ADDRESS/(2^8)));
      | REGISTER_ADDRESS_LSB = uint8(rem(REGISTER_ADDRESS,2^8));
  wires:
  Constant1/1 -> I2C WRITE: SYSRANGE_START/1(DATA)

== system TEST_TCP/HARDWARE/SENSORS/WALL RANGE SENSOR/VL6180X_I2C_FRONT/VL6180X INITIALIZATION/CHECK INITIALIZATION ==
  Compare To Constant1 : simulink/Logic and Bit Operations/Compare To Constant  relop===  const=hex2dec('1F')  OutDataTypeStr=boolean
  Compare To Constant2 : simulink/Logic and Bit Operations/Compare To Constant  relop===  const=hex2dec('31')  OutDataTypeStr=boolean
  Compare To Constant3 : simulink/Logic and Bit Operations/Compare To Constant  relop===  const=hex2dec('00')  OutDataTypeStr=boolean
  Compare To Constant4 : simulink/Logic and Bit Operations/Compare To Constant  relop===  const=hex2dec('63')  OutDataTypeStr=boolean
  Compare To Constant5 : simulink/Logic and Bit Operations/Compare To Constant  relop===  const=hex2dec('24')  OutDataTypeStr=boolean
  Demux : Demux  Outputs=2
  I2C READ: SYSALS_INTEGRATION_PERIOD : Subsystem  mask{SLAVE_ADDRESS=VL6180X.ADDRESS, REGISTER_ADDRESS=VL6180X.SYSALS_INTEGRATION_PERIOD, N=2}
      mask prompts: SLAVE_ADDRESS "SLAVE ADDRESS"; REGISTER_ADDRESS "REGISTER ADDRESS"; N "NUMBER OF DATA (bytes)"
  I2C READ: SYSRANGE_MAX_CONVERGENCE_TIME : Subsystem  mask{SLAVE_ADDRESS=VL6180X.ADDRESS, REGISTER_ADDRESS=VL6180X.SYSRANGE_MAX_CONVERGENCE_TIME, N=1}
      mask prompts: SLAVE_ADDRESS "SLAVE ADDRESS"; REGISTER_ADDRESS "REGISTER ADDRESS"; N "NUMBER OF DATA (bytes)"
  "I2C READ: 0x1A7 " : Subsystem  mask{SLAVE_ADDRESS=VL6180X.ADDRESS, REGISTER_ADDRESS=hex2dec('1A7'), N=1}
      mask prompts: SLAVE_ADDRESS "SLAVE ADDRESS"; REGISTER_ADDRESS "REGISTER ADDRESS"; N "NUMBER OF DATA (bytes)"
  I2C WRITE: SYSTEM_INTERRUPT_CONFIG_GPIO : Subsystem  mask{SLAVE_ADDRESS=VL6180X.ADDRESS, REGISTER_ADDRESS=VL6180X.SYSTEM_INTERRUPT_CONFIG_GPIO, N=1}
      mask prompts: SLAVE_ADDRESS "SLAVE ADDRESS"; REGISTER_ADDRESS "REGISTER ADDRESS"; N "NUMBER OF DATA (bytes)"
  Logical Operator : Logic  Inputs=5  IconShape=distinctive  AllPortsSameDT=off  OutDataTypeStr=boolean
  STATUS : Outport  VectorParamsAs1DForOutWhenUnconnected=off
  wires:
  Demux/2 -> Compare To Constant4/1
  "I2C READ: 0x1A7 "/1(DATA) -> Compare To Constant1/1
  Compare To Constant2/1 -> Logical Operator/5
  Demux/1 -> Compare To Constant3/1
  I2C READ: SYSRANGE_MAX_CONVERGENCE_TIME/1(DATA) -> Compare To Constant2/1
  I2C READ: SYSALS_INTEGRATION_PERIOD/1(DATA) -> Demux/1
  I2C WRITE: SYSTEM_INTERRUPT_CONFIG_GPIO/1(DATA) -> Compare To Constant5/1
  Compare To Constant5/1 -> Logical Operator/4
  Compare To Constant1/1 -> Logical Operator/1
  Compare To Constant4/1 -> Logical Operator/3
  Compare To Constant3/1 -> Logical Operator/2
  Logical Operator/1 -> STATUS/1

== system TEST_TCP/HARDWARE/SENSORS/WALL RANGE SENSOR/VL6180X_I2C_FRONT/VL6180X INITIALIZATION/I2C READ: SYSTEM_FRESH_OUT_OF_RESET ==
  Constant : Constant  Value=REGISTER_ADDRESS  OutDataTypeStr=uint16  SampleTime=SAMPLING_TIME
  DATA TO BE READ : raspberrypiCommlib/I2C Master Read  Priority=20  BoardProperty=Pi 3 Model B+  Mode=Master  SlaveAddress=SLAVE_ADDRESS  SlaveByteOrder=BigEndian  Direction=Receiver  RegisterAddressMode=off  RegisterAddress=0  SlaveDataType=uint8  DataLength=uint8(N)  NoAck=off  RepeatedStart=off  OutputStatus=off  SampleTime=SAMPLING_TIME
  REGISTER ADDRESS : raspberrypiCommlib/I2C Master Write  Priority=10  BoardProperty=Pi 3 Model B+  Mode=Master  SlaveAddress=SLAVE_ADDRESS  SlaveByteOrder=BigEndian  Direction=Transmitter  RegisterAddressMode=off  RegisterAddress=hex2dec('207')  SlaveDataType=uint8  DataLength=1  NoAck=off  RepeatedStart=off  OutputStatus=off
  DATA : Outport  VectorParamsAs1DForOutWhenUnconnected=off
  wires:
  Constant/1 -> REGISTER ADDRESS/1
  DATA TO BE READ/1 -> DATA/1
